simulink model "Simulation"  (R2019b)
settings: Solver=ode45  StartTime=0.0  StopTime=40  MaxStep=0.2  RelTol=1e-3  EnableMultiTasking=on
model workspace (MAT data in the model file):
  g_density = 5
libraries: sm_stewart_platform_lib x8, sm_lib x2, nesl_utility x1
Description:
  | Stewart Platform
  | 
  | This model shows a Stewart platform manipulator that can track a
  | parameterized reference trajectory. The shape, size, and kinematics of
  | the manipulator are highly configurable.
  | 
  | The reference trajectory is
  | specified in 6-D pose space, and an inverse kinematics module
  | converts it into one through 6-D leg position space.  A generic PID
  | controller attempts to drive the manipulator along the desired
  | trajectory.
settings Model: FPTRunName=Active  Creator=MathWorks  LastModifiedBy=hakon
settings DataIOCC: LimitDataPoints=on  SaveFormat=Array  SignalLoggingSaveFormat=ModelDataLogs  ReturnWorkspaceOutputs=off
settings OptimizationCC: ExpressionDepthLimit=2147483647  LifeSpan=inf
settings DebuggingCC: UnderspecifiedInitializationDetection=Classic  MergeDetectMultiDrivingBlocksExec=none  SolverPrmCheckMsg=warning  FcnCallInpInsideContextMsg=warning  StateNameClashWarn=warning  SFUnexpectedBacktrackingDiag=warning  SFNoUnconditionalDefaultTransitionDiag=warning  SFExecutionAtInitializationDiag=none  ArithmeticOperatorsInVariantConditions=warning
settings HardwareCC: ProdBitPerPointer=32  ProdBitPerSizeT=32  ProdBitPerPtrDiffT=32  ProdLargestAtomicFloat=None  ProdIntDivRoundTo=Undefined  ProdEndianess=Unspecified  ProdWordSize=32  ProdHWDeviceType=32-bit Generic
settings ModelReferenceCC: PropagateSignalLabelsOutOfModel=off
settings SFSimCC: SimUseLocalCustomCode=off  CustomCodeUndefinedFunction=UseInterfaceOnly
settings RTWCC: RTWUseLocalCustomCode=off
settings CodeAppCC: StateflowObjectComments=on
settings GRTTargetCC: TargetLangStandard=C89/C90 (ANSI)  GeneratePreprocessorConditionals=Disable all  CombineOutputUpdateFcns=off  GRTInterface=on
settings ConfigComp: CovMetricSettings=dw  CovHtmlReporting=on  CovSaveCumulativeToWorkspaceVar=on  CovSaveSingleToWorkspaceVar=on  CovExternalEMLEnable=off
settings SimscapeCC: SimscapeNormalizeSystem=off  SimscapeLogDataHistory=15000
settings ConfigurationSet: Description=SimMechanics 2G

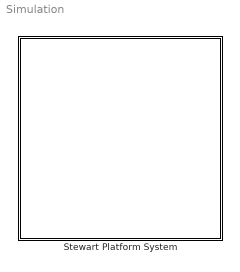
== system Simulation ==
  Stewart Platform System : Subsystem  mask(Stewart Platform System){base_rad=30, base_thick=5, platform_rad=20, platform_thick=0.5, hex_skew=-0.25, upper_leg_len=8, lower_leg_len=8, leg_rad=2, collar_thick=0.5, gripper_height=30, claw_length=8, claw_width=3, claw_thick=1, end_eff_base_thick=2, flange_len=2.3, flange_width=1.75, flange_thick=.8, ic_R=eye(3), ic_d=[0 0 15]', Kp=600, Ki=60, Kd=10}
      mask prompts: base_rad "Base Radius  (cm)"; base_thick "Base Thickness (cm)"; platform_rad "Platform Radius (cm)"; platform_thick "Platform Thickness (cm)"; hex_skew "Hexagon Skew"; upper_leg_len "Upper Leg Length (cm)"; lower_leg_len "Lower Leg Length (cm)"; leg_rad "Leg Radius (cm)"; collar_thick "Collar Thickness (cm)"; gripper_height "Gripper Height (cm)"; claw_length "Claw Length (cm)"; claw_width "Claw Width (cm)"; claw_thick "Claw Thickness (cm)"; end_eff_base_thick "Base Thickness (cm)"; flange_len "Flange Length (cm)"; flange_width "Flange Width (cm)"; flange_thick "Flange Thickness (cm)"; ic_R "Rotation Matrix [3 x 3]"; ic_d "Displacement Vector (cm) [3 x 1]"; Kp "Controller Proportional Gain (N / cm)"; Ki "Controller Integral Gain (N / (cm s))"; Kd "Controller Derivative Gain (N / (cm / s)))"
      mask help:
      | Models a complete Stewart platform manipulator system.  The system can be driven to position and orient a special gripper frame according to specified trajectories.
      |
      | The system comprises a mechanical manipulator, an inverse kinematics module, and a control system.
      mask init:
      | params = struct( ...
      |     'base_thick',        base_thick,     ...
      |     'base_radius',       base_rad,       ...
      |     'platform_thick',    platform_thick, ...
      |     'platform_radius',   platform_rad,   ...
      |     'skew',              hex_skew,       ...
      |     'flange_length',     flange_len,     ...
      |     'flange_width',      flange_width,   ...
      |     'flange_thick',      flange_thick,   ...
      |     'leg_radius',        leg_rad,        ...
      |     'upper_leg_length',  upper_leg_len,  ...
      |     'lower_leg_length',  lower_leg_len,  ...
      |     'gripper_height',    gripper_height  ...
      |     );
      | 
      | [B, P, nom_length] = sm_stewart_platform_setup(params);
      | 
      | lengths = sm_stewart_platform_ik(B, P, nom_length, ic_R, ic_d);
      mask Help:
      | A <em>Stewart Platform System</em> models a complete Stewart platform manipulator system.  The system can be driven to position and orient a special gripper frame according to specified trajectories.
      | 
      | <h3>Subsystems</h3>
      | 
      | A Stewart platform system comprises three primary subsystems:
      | 
      | <ol>
      | 
      | <li><b>Manipulator</b> The manipulator is the Simscape Multibody subsystem describing the mechanical structure of the Stewart platform.  The manipulator contains two hexagonal plates, a lower base plate and an upper platform plate, connected by six articulated legs.  The base plate is anchored to the world frame, and the platform plate is controlled to position and orient the gripper frame. The manipulator component provides sensing and actuation signals to interface to a controller.
      | 
      |   The manipulator is highly parameterized.  Most parameters of the Stewart platform system are physical lengths and other parameters that control the shapes and sizes of the components of the manipulator. By varying these parameters, a wide range of Stewart platform manipulators can be realized.
      | 
      | <li><b>Inverse Kinematics (IK) Module</b> The inverse kinematics module is a pure Simulink subsystem that maps time-varying signals describing the desired position and orientation of the gripper frame into time-varying scalar signals specifying the positions and velocities of the prismatic primitives of the leg joints.  This is an essential component of a complete Stewart platform system because the user of the system typically expresses a desired trajectory in the 6-D space of positions and orientations of the gripper frame, but the manipulator control is simplest in the 6-D space of leg joint positions. The IK module forms the bridge between these two spaces.
      | 
      |   The mathematics performed within the IK module is heavily dependent on the physical parameters that determine the shape and size of the manipulator itself.  Most of the parameters that govern the manipulator are also used within the IK module.
      | 
      | <li><b>Control System</b> The control system is a pure Simulink subsystem that attempts to drive the gripper frame along its desired trajectory by controlling the positions of the prismatic primitives of the leg joints. It uses a standard PID control scheme, with gains specified by Stewart platform system parameters.  The control uses no information about the forward or inverse kinematics of the platform; it simply tries to drive a point along a trajectory in 6-D space.
      | 
      |   The controller takes both the desired and actual leg position vectors and the first derivatives of these quantities.  It generates a 6-D commanded force output that can be used to drive the six leg lengths to thei desired values.
      | 
      |   Because the size and shape of the Stewart platform manipulator can vary significantly depending on the parameter settings, the controller gains may need to be adjusted in order to control the manipulator to the desired trajectory.
      | 
      | </ol>
      | 
      | <h3>Base and Platform Plates</h3>
      | 
      | The <em>Plates</em> tab parameters specify the geometry of the base and platform hexagon plates of the Stewart platform manipulator.  See the documentation of the <em>Hexagon Plate</em> library block for details.
      | 
      | <ul>
      | 
      | <li> <b>Base Radius</b> The radius of the base plate.  The vertices of the hexagonal cross section all lie on a circle of this radius.
      | 
      | <li> <b>Base Thickness</b> The thickness of the base plate.
      | 
      | <li> <b>Platform Radius</b> The radius of the platform plate.  The vertices of the hexagonal cross section all lie on a circle of this radius.
      | 
      | <li> <b>Platform Thickness</b> The thickness of the platform plate.
      | 
      | <li> <b>Hexagon Skew</b> The common skew factor of the base and platform plates. This value, in the range (-0.5, +0.5), determines the shape of the three-fold symmetric hexagons.  A zero skew factor produces regular hexagons.  As the skew factor magnitude increases, the hexagons become more triangular.
      | 
      | </ul>
      | 
      | <h3>Legs</h3>
      | 
      | The <em>Legs</em> tab parameters specify the common geometry of the six legs of the Stewart platform manipulator.  See the documentation of the <em>Leg</em> library block for details.
      | 
      | <ul>
      | 
      | <li> <b>Upper Leg Length</b> The length of the upper leg, including its end collars.
      | 
      | <li> <b>Lower Leg Length</b> The length of the lower leg, including its end collars.
      | 
      | <li> <b>Leg Radius</b> The common radius of the upper and lower leg segments. Each segment's cross section is a regular hexagon inscribed in a circle of this radius.
      | 
      | <li> <b>Collar Thickness</b> The thickness of the hexagonal collars adjoined to the ends of each leg segment.
      | 
      | </ul>
      | 
      | <h3>End Effector</h3>
      | 
      | The <em>End Eff</em> tab parameters specify the geometry of the end effector attached to the platform plate of the Stewart platform manipulator. See the documentation of the <em>End Effector</em> block within the <em>Manipulator</em> subsystem for details.
      | 
      | <ul>
      | 
      | <li> <b>Gripper Height</b> The vertical distance from the origin of the gripper frame to the top surface of the movable platform plate.
      | 
      | <li> <b>Claw Length</b> The length (height) of the trapezoidal claws of the gripper.
      | 
      | <li> <b>Claw Width</b> The width of the trapezoidal claws of the gripper where they attach to the gripper base.
      | 
      | <li> <b>Claw Thickness</b> The thickness of the trapezoidal claws of the gripper.
      | 
      | <li> <b>Base Thickness</b> The thickness of the triangular gripper base.
      | 
      | </ul>
      | 
      | <h3>Flanges</h3>
      | 
      | The <em>Flanges</em> tab parameters specify the common geometry of the 48 flanges attached to the hexagonal plates and legs of the Stewart platform manipulator.  Each of the 12 universal joints is supported by four flanges.  See the documentation of the <em>Flange</em> library block for details.
      | 
      | <ul>
      | 
      | <li> <b>Flange Length</b> The length of the rectangular prism portion of the flanges.
      | 
      | <li> <b>Flange Width</b> The width of the rectangular prism portion of the flanges.
      | 
      | <li> <b>Flange Thickness</b> The thickness of the flanges.
      | 
      | </ul>
      | 
      | <h3>Initial Conditions</h3>
      | 
      | The <em>IC</em> tab parameters specify the initial conditions of the Stewart Platform manipulator for simulation.  Specifically, these specify the <em>position</em> of the manipulator; the simulation always starts from a rest (zero velocity) state.
      | 
      | The initial position is defined by specifying pose of the gripper frame relative to the world frame.  This is typically a convenient parameterization for a user of the manipulator.  The world frame is also the reference frame of the manipulator base plate.  This is a frame with origin at the center of the manipulator base (which is in its interior), and with z-axis pointed directly upward.
      | 
      | An Update Diagram (Ctrl-D) operation will attempt to assemble the manipulator in the specified initial position.  Some initial positions may be incompatible with the kinematics of the manipulator, based on other parameter settings.  In such cases, the assembly will fail.
      | 
      | Also note that if the initial position differs significantly from the desired trajectory (specified through the input signal ports) at time zero, the manipulator's motion may be subject to large transients at the start of simulation.
      | 
      | <ul>
      | 
      | <li> <b>Rotation Matrix</b> The rotation matrix mapping directions in the gripper frame to directions in the world frame.  This should be a 3 x 3 orthogonal matrix determinant +1.  The columns of this matrix are the canonical i, j, and k unit vectors of the gripper frame resolved in world frame coordinates.
      | 
      | <li> <b>Displacement Vector</b> The location of the origin of the gripper frame in world frame coordinates.  This should be a 3 x 1 column vector.  The z-coordinate should generally be positive, on the order of the nominal lengths of the legs.
      | 
      | </ul>
      | 
      | If the rotation matrix is the identity and the x- and y-coordinates of the displacement vector are zero, the initial configuration of the manipulator will be symmetric with all leg positions equal.
      | 
      | <h3>Controller Gains</h3>
      | 
      | The <em>Control</em> tab parameters specify the gains of the internal controller used to control the manipulator's pose according to a specified trajectory.  The controller uses a generic PID control scheme.  The gains may need to be adjusted to be appropriate if the parameters governing the size and kinematics of the manipulator are changed significantly.
      | 
      | See the documentation of the <em>Controller</em> subsystem for details.
      | 
      | <ul>
      | 
      | <li> <b>Controller Proportional Gain</b> The proportional (P) gain of the internal PID controller.
      | 
      | <li> <b>Controller Integral Gain</b> The integral (I) gain of the internal PID controller.
      | 
      | <li> <b>Controller Derivative Gain</b> The derivative (D) gain of the internal PID controller.
      | 
      | </ul>
      | 
      | 
      | 
      | <h3>Ports</h3>
      | 
      | <ul>
      | 
      | <li><b>d</b> The desired displacement vector of the gripper frame relative to the world frame as a signal input.  This value should be a 3 x 1 vector in units of centimeters.  It specifies the desired origin of the gripper frame in world frame coordinates as a function of time.  This signal is analogous to the <em>Displacement Vector</em> on the <em>IC</em> parameter tab.
      | 
      | <li><b>R</b> The desired rotation matrix from the gripper frame to the world frame as a signal input.  This value should be a 3 x 3 orthogonal matrix with +1 determinant.  The columns of this matrix are the canonical i, j, and k unit vectors of the gripper frame resolved in world frame coordinates, specified as functions of time.  This signal is analogous to the <em>Rotation Matrix</em> on the <em>IC</em> parameter tab.
      | 
      | <li><b>d'</b> The first time derivative of the desired displacement vector of the gripper frame relative to the world frame as a signal input.  This value should be the first time derivative of the signal provided on the <em>d</em> port: a 3 x 1 vector in units of centimeters/second. It specifies the velocity of the origin of the gripper frame in  world frame coordinates as a function of time.
      | 
      | <li><b>R'</b> The first time derivative of the desired rotation matrix from the gripper frame to the world frame as a signal input.  This value should be the first time derivative of the signal provided on the <em>R</em> port: a 3 x 3 matrix.
      | 
      | <li><b>Pos</b> The position of the gripper with respect to the world frame as a 3 x 1 position vector in units of centimeters.
      | </ul>
      | 
      | <!--  LocalWords:  Eff IC Ctrl IK
      |  -->
      mask Display:
      | image(imread('sm_stewart_platform_system.png'))
      | color('yellow')
      | port_label('Input', 1, 'd')
      | port_label('Input', 2, 'R')
      | port_label('Input', 3, 'd''')
      | port_label('Input', 4, 'R''')
      | port_label('Output', 1, 'Pos')

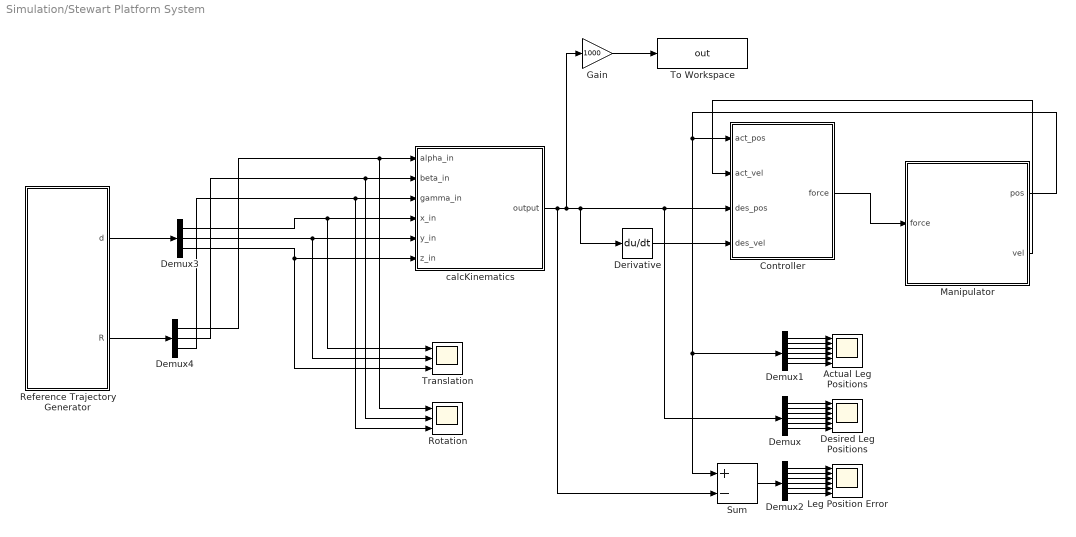
== system Simulation/Stewart Platform System ==
  Actual Leg Positions : Scope  NumInputPorts=6
  Controller : Subsystem  mask(PID Controller){Kp=Kp, Ki=Ki, Kd=Kd}
      mask prompts: Kp "Proportional Gain"; Ki "Integral Gain"; Kd "Derivative Gain"
      mask help:
      | Generates an actuation output based on a desired trajectory and an actual trajectory, using a generic proportional-integral-derivative (PID) control law.  The three control gains are specified through parameters.
      |
      | Both the desired and actual trajectories are specified by separate position and velocity input signals.  The controller is generic and can control to trajectories through state spaces of arbitrary dimension; the only requirement is that all four inputs have the same dimension.
      mask Help:
      | A <em>PID Controller</em> generates an actuation output based on a desired trajectory and an actual trajectory, using a generic proportional-integral-derivative (PID) control law.  The three control gains are specified through parameters.
      | 
      | Both the desired and actual trajectories are specified by separate position and velocity input signals.  The controller is generic and can control to trajectories through state spaces of arbitrary dimension; the only requirement is that all four inputs have the same dimension.
      | 
      | This block is not specific to the Stewart platform and could serve in any general purpose control library.  For the Stewart platform application, the trajectories are all through the 6-D leg-position space.
      | 
      | <h3>Gains</h3>
      | 
      | The parameters specify the gains of the controller.
      | 
      | <ul>
      | 
      | <li> <b>Proportional Gain</b> The gain that determines the strength of the control actuation in response to current deviations between actual and desired positions.  This affects the responsiveness of the controller but can lead to instability if set too high.
      | 
      | <li> <b>Integral Gain</b> The gain that determines the strength of the control actuation in response to deviations between actual and desired positions that persist over time.  A nonzero integral term is often necessary to avoid <em>droop</em> (steady-state error).  Higher values reduce the transient response of the controller but can cause overshoot in the controlled position.
      | 
      | <li> <b>Derivative Gain</b> The gain that determines the strength of the control actuation in response to the derivative of the deviations between actual and desired positions.  This is a damping component used to reduce overshoot in the controlled position; the tradeoff is that it reduces the transient response of the controller.  Higher values increase the stiffness of the system and can lead to instability.
      | 
      | </ul>
      | 
      | 
      | <h3>Ports</h3>
      | 
      | <ul>
      | 
      | <li> <b>act_pos</b> The current actual position of the plant.
      | 
      | <li> <b>act_pos</b> The current actual velocity of the plant.  This should be the time derivative of the <em>act_pos</em> signal.
      | 
      | <li> <b>des_pos</b> The current desired position of the plant.
      | 
      | <li> <b>des_pos</b> The current desired velocity of the plant.  This should be the time derivative of the <em>des_pos</em> signal.
      | 
      | </ul>
  Demux : Demux  Outputs=6
  Demux1 : Demux  Outputs=6
  Demux2 : Demux  Outputs=6
  Demux3 : Demux  Outputs=3
  Demux4 : Demux  Outputs=3
  Derivative : Derivative
  Desired Leg Positions : Scope  NumInputPorts=6
  Gain : Gain  Gain=1000
  Leg Position Error : Scope  NumInputPorts=6
  Manipulator : Subsystem  mask(Stewart Platform Manipulator){}
      mask help: Models the mechanical portion of a complete Stewart platform manipulator system: the manipulator itself. Almost all of the Simscape Multibody blocks of the full system are contained in the manipulator subsystem.
      mask Help:
      | A <em>Stewart Platform Manipulator</em> models the mechanical portion of a complete Stewart platform manipulator system: the manipulator itself.  Almost all of the Simscape Multibody blocks of the full system are contained in the manipulator subsystem.
      | 
      | The manipulator subsystem exposes two frames: the world frame, to which the base is anchored, and the gripper frame, which is the frame at the distil end of the end effector.  Typically, a user wants to control the manipulator transformation, which is the 3-D rigid transformation from the gripper frame to the world frame.
      | 
      | The manipulator subsystem has no internal control.  However, it reports the positions and velocities of the prismatic primitives of all six cylindrical leg joints as output signals and takes the actuation forces to be applied to these primitives as input signals.  When connected to an appropriate controller, these signals are sufficient to provide any of a variety of control schemes for the manipulator.
      | 
      | <h3>Parameterization</h3>
      | 
      | The manipulator is highly parameterized.  Most of the physical dimensions of its component pieces can be controlled via parameters.  These parameters are all defined in the containing <em>Stewart Platform System</em>.  The manipulator's parameters are inherited from that block; they are not defined explicitly in this block's mask.  The parameters are also needed for the <em>Stewart Platform Inverse Kinematics</em> block.
      | 
      | See the documentation of the <em>Stewart Platform System</em> block for details.
      | 
      | <h3>Ports</h3>
      | 
      | <ul>
      | 
      | <li> <b>gripper</b> The gripper frame.  This frame is fixed at the distil end of the end effector attached to the platform plate of the Stewart platform manipulator.  It is identified with a frame glyph in the visualization of the manipulator.  Typically, a user of the manipulator wants to control the pose of this frame, with respect to a reference frame such as world.
      | 
      | <li> <b>world</b> The world frame.  This is also the reference frame of the base plate of the Stewart platform manipulator, which is rigidly attached to the world frame.
      | 
      | <li><b>pos</b> The positions of the prismatic primitives of the six leg joints as a 6 x 1 output signal in units of centimeters.
      | 
      | <li><b>vel</b> The velocities of the prismatic primitives of the six leg joints as a 6 x 1 output signal in units of centimeters/second.
      | 
      | <li><b>force</b> The actuation forces applied to the prismatic primitives of the six leg joints as a 6 x 1 input signal in units of Newtons.
      | 
      | </ul>
      | 
      | <!--  LocalWords:  Eff IC Ctrl pos vel
      |  -->
      mask Display:
      | image(imread('sm_stewart_platform_manipulator.png'))
      | color('white')
      | port_label('LConn', 1, 'world')
      | port_label('RConn', 1, 'gripper')
      | color('yellow')
      | port_label('Input', 1, 'force')
      | port_label('Output', 1, 'pos')
      | port_label('Output', 2, 'vel')
  Reference Trajectory Generator : Subsystem
  Rotation : Scope  NumInputPorts=3
  Sum : Sum  Inputs=+-
  To Workspace : ToWorkspace  VariableName=out  SaveFormat=Timeseries  SampleTime=-1
  Translation : Scope  NumInputPorts=3
  calcKinematics : MATLAB Function  TreatAsAtomicUnit=on
  wires:
  Manipulator/2(vel) -> Controller/2(act_vel)
  Demux/1 -> Desired Leg Positions/1
  Demux/2 -> Desired Leg Positions/2
  Demux/3 -> Desired Leg Positions/3
  Demux/4 -> Desired Leg Positions/4
  Demux/5 -> Desired Leg Positions/5
  Demux/6 -> Desired Leg Positions/6
  Demux1/1 -> Actual Leg Positions/1
  Demux1/2 -> Actual Leg Positions/2
  Demux1/3 -> Actual Leg Positions/3
  Demux1/4 -> Actual Leg Positions/4
  Demux1/5 -> Actual Leg Positions/5
  Demux1/6 -> Actual Leg Positions/6
  Demux2/1 -> Leg Position Error/1
  Demux2/2 -> Leg Position Error/2
  Demux2/3 -> Leg Position Error/3
  Demux2/4 -> Leg Position Error/4
  Demux2/5 -> Leg Position Error/5
  Demux2/6 -> Leg Position Error/6
  Sum/1 -> Demux2/1
  Controller/1(force) -> Manipulator/1(force)
  Manipulator/1(pos) -> Controller/1(act_pos), Demux1/1, Sum/1
  calcKinematics/1(output) -> Sum/2, Gain/1, Derivative/1, Demux/1, Controller/3(des_pos)
  Derivative/1 -> Controller/4(des_vel)
  Reference Trajectory Generator/1(d) -> Demux3/1
  Demux3/2 -> Translation/2, calcKinematics/5(y_in)
  Demux3/3 -> Translation/3, calcKinematics/6(z_in)
  Reference Trajectory Generator/2(R) -> Demux4/1
  Demux4/1 -> Rotation/1, calcKinematics/1(alpha_in)
  Demux4/2 -> Rotation/2, calcKinematics/2(beta_in)
  Demux4/3 -> Rotation/3, calcKinematics/3(gamma_in)
  Demux3/1 -> Translation/1, calcKinematics/4(x_in)
  Gain/1 -> To Workspace/1

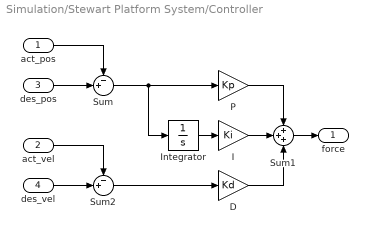
== system Simulation/Stewart Platform System/Controller ==
  act_pos : Inport
  act_vel : Inport  Port=2
  des_pos : Inport  Port=3
  des_vel : Inport  Port=4
  D : Gain  Gain=Kd  SaturateOnIntegerOverflow=on  OutDataTypeStr=Inherit: Same as input  ParamDataTypeStr=Inherit: Same as input
  I : Gain  Gain=Ki  SaturateOnIntegerOverflow=on  OutDataTypeStr=Inherit: Same as input  ParamDataTypeStr=Inherit: Same as input
  Integrator : Integrator  ZeroCross=off
  P : Gain  Gain=Kp  SaturateOnIntegerOverflow=on  OutDataTypeStr=Inherit: Same as input  ParamDataTypeStr=Inherit: Same as input
  Sum : Sum  Inputs=-+|  SaturateOnIntegerOverflow=on  InputSameDT=on  OutDataTypeStr=Inherit: Same as first input
  Sum1 : Sum  Inputs=+++  SaturateOnIntegerOverflow=on  InputSameDT=on  OutDataTypeStr=Inherit: Same as first input
  Sum2 : Sum  Inputs=-+|  SaturateOnIntegerOverflow=on  InputSameDT=on  OutDataTypeStr=Inherit: Same as first input
  force : Outport  VectorParamsAs1DForOutWhenUnconnected=off
  wires:
  Sum2/1 -> D/1
  D/1 -> Sum1/3
  Integrator/1 -> I/1
  P/1 -> Sum1/1
  I/1 -> Sum1/2
  Sum/1 -> P/1, Integrator/1
  act_pos/1 -> Sum/1
  des_pos/1 -> Sum/2
  Sum1/1 -> force/1
  act_vel/1 -> Sum2/1
  des_vel/1 -> Sum2/2

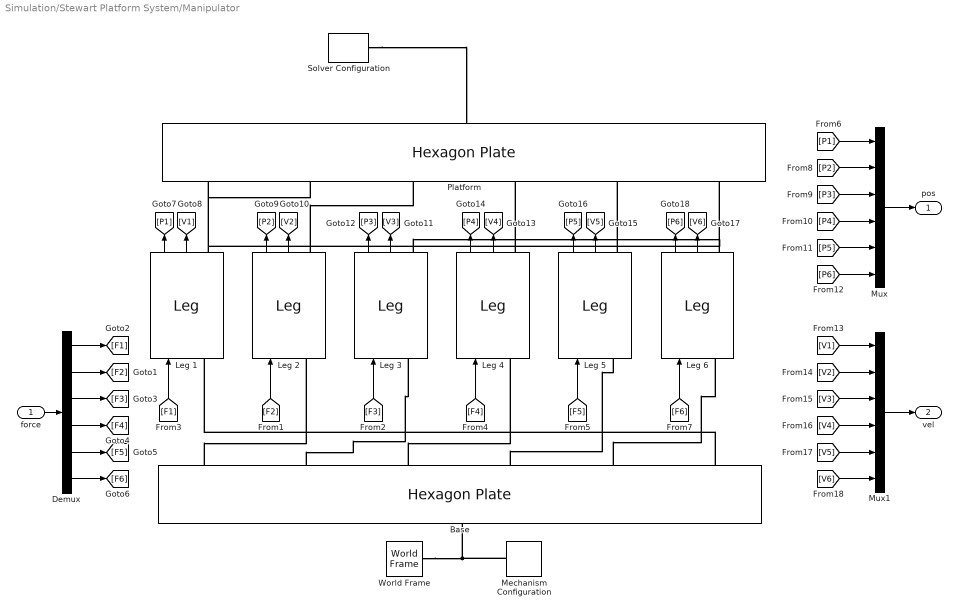
== system Simulation/Stewart Platform System/Manipulator ==
  force : Inport
  Base : sm_stewart_platform_lib/Hexagon Plate  kind=base  hex_rad=base_rad  hex_thick=base_thick  hex_skew=hex_skew  flange_sep=2 * leg_rad * cos(pi/6) - flange_thick  flange_len=flange_len  flange_width=flange_width  flange_thick=flange_thick  diffuse=[0.4 0.3 0.2 0.5]  specular=[0 0 0]  shininess=10
      settings: SourceProductName=Simscape Multibody  SourceProductBaseCode=MS
  Demux : Demux  Outputs=6
  Leg 1 : sm_stewart_platform_lib/Leg  upper_leg_len=upper_leg_len  lower_leg_len=lower_leg_len  rad=leg_rad  collar_thick=collar_thick  flange_len=flange_len  flange_width=flange_width  flange_thick=flange_thick  asm_offset=lengths(1)
      settings: SourceProductName=Simscape Multibody  SourceProductBaseCode=MS
  Leg 2 : sm_stewart_platform_lib/Leg  upper_leg_len=upper_leg_len  lower_leg_len=lower_leg_len  rad=leg_rad  collar_thick=collar_thick  flange_len=flange_len  flange_width=flange_width  flange_thick=flange_thick  asm_offset=lengths(2)
      settings: SourceProductName=Simscape Multibody  SourceProductBaseCode=MS
  Leg 3 : sm_stewart_platform_lib/Leg  upper_leg_len=upper_leg_len  lower_leg_len=lower_leg_len  rad=leg_rad  collar_thick=collar_thick  flange_len=flange_len  flange_width=flange_width  flange_thick=flange_thick  asm_offset=lengths(3)
      settings: SourceProductName=Simscape Multibody  SourceProductBaseCode=MS
  Leg 4 : sm_stewart_platform_lib/Leg  upper_leg_len=upper_leg_len  lower_leg_len=lower_leg_len  rad=leg_rad  collar_thick=collar_thick  flange_len=flange_len  flange_width=flange_width  flange_thick=flange_thick  asm_offset=lengths(4)
      settings: SourceProductName=Simscape Multibody  SourceProductBaseCode=MS
  Leg 5 : sm_stewart_platform_lib/Leg  upper_leg_len=upper_leg_len  lower_leg_len=lower_leg_len  rad=leg_rad  collar_thick=collar_thick  flange_len=flange_len  flange_width=flange_width  flange_thick=flange_thick  asm_offset=lengths(5)
      settings: SourceProductName=Simscape Multibody  SourceProductBaseCode=MS
  Leg 6 : sm_stewart_platform_lib/Leg  upper_leg_len=upper_leg_len  lower_leg_len=lower_leg_len  rad=leg_rad  collar_thick=collar_thick  flange_len=flange_len  flange_width=flange_width  flange_thick=flange_thick  asm_offset=lengths(6)
      settings: SourceProductName=Simscape Multibody  SourceProductBaseCode=MS
  Mechanism Configuration : sm_lib/Utilities/Mechanism Configuration  UniformGravity=Constant  GravityVector=[0 0 -9.81]  GravityUnits=m/s^2  LinearizationDelta=0.001
  Mux : Mux  Inputs=6
  Mux1 : Mux  Inputs=6
  Platform : sm_stewart_platform_lib/Hexagon Plate  kind=platform  hex_rad=platform_rad  hex_thick=platform_thick  hex_skew=hex_skew  flange_sep=2 * leg_rad * cos(pi/6) - flange_thick  flange_len=flange_len  flange_width=flange_width  flange_thick=flange_thick  diffuse=[.7 .7 .3 0.75]  specular=[.7 .7 .3 0.75]  shininess=90
      settings: SourceProductName=Simscape Multibody  SourceProductBaseCode=MS
  Solver Configuration : nesl_utility/Solver Configuration  PhysicalDomain=network_engine_domain  SubClassName=solver  LeftPortType=input  RightPortType=generic  Tones=[]  Harmonics=[]  SimulateNoise=off  Profile=off  UseLocalSampling=off  EnableSwitchedLinearOptims=on  FrequencyDomain=off  UseCCode=off  RelTol=0.001  AbsTol=1e-06  MinStep=1e-09  ToWorkspace=off  RevertToSquareIcSolve=off  NumHomotopyIterations=100  PhasorMode=off  PhasorModeNumHarmonics=1  DoDC=off  ResidualTolerance=1e-9  UseLocalSolver=off  LocalSolverChoice=NE_BACKWARD_EULER_ADVANCER  LocalSolverSampleTime=.001  DoFixedCost=off  MaxNonlinIter=3  MaxModeIter=2  LinearAlgebra=Sparse  EquationFormulation=NE_TIME_EF  DelaysMemoryBudget=1024  AutomaticFiltering=on  FilteringTimeConstant=0.001  PartitionStorageMethod=AS_NEEDED  PartitionMemoryBudget=1024  PartitionMethod=FAST
  World Frame : sm_lib/Frames and Transforms/World Frame
  pos : Outport  VectorParamsAs1DForOutWhenUnconnected=off
  vel : Outport  Port=2  VectorParamsAs1DForOutWhenUnconnected=off
  wires:
  Demux/1 -> [F1]
  Demux/2 -> [F2]
  Demux/3 -> [F3]
  Demux/4 -> [F4]
  Demux/5 -> [F5]
  Demux/6 -> [F6]
  [F1] -> Leg 1/1
  [F2] -> Leg 2/1
  [F3] -> Leg 3/1
  [F4] -> Leg 4/1
  [F5] -> Leg 5/1
  [F6] -> Leg 6/1
  force/1 -> Demux/1
  Leg 1/1 -> [P1]
  Leg 1/2 -> [V1]
  Leg 2/1 -> [P2]
  Leg 2/2 -> [V2]
  Leg 3/1 -> [P3]
  Leg 3/2 -> [V3]
  Leg 4/1 -> [P4]
  Leg 4/2 -> [V4]
  Leg 5/1 -> [P5]
  Leg 5/2 -> [V5]
  Leg 6/1 -> [P6]
  Leg 6/2 -> [V6]
  Mux/1 -> pos/1
  [P1] -> Mux/1
  [P2] -> Mux/2
  [P3] -> Mux/3
  [P4] -> Mux/4
  [P5] -> Mux/5
  [P6] -> Mux/6
  [V1] -> Mux1/1
  [V2] -> Mux1/2
  [V3] -> Mux1/3
  [V4] -> Mux1/4
  [V5] -> Mux1/5
  [V6] -> Mux1/6
  Mux1/1 -> vel/1
  connections:
  Solver Configuration/RConn1 -- Platform/LConn1
  Mechanism Configuration/RConn1 -- World Frame/RConn1 -- Base/LConn1
  Base/RConn1 -- Leg 2/LConn1
  Base/RConn2 -- Leg 3/LConn1
  Base/RConn3 -- Leg 4/LConn1
  Base/RConn4 -- Leg 5/LConn1
  Base/RConn5 -- Leg 6/LConn1
  Base/RConn6 -- Leg 1/LConn1
  Leg 1/RConn1 -- Platform/RConn2
  Leg 2/RConn1 -- Platform/RConn3
  Leg 3/RConn1 -- Platform/RConn4
  Leg 4/RConn1 -- Platform/RConn5
  Leg 5/RConn1 -- Platform/RConn6
  Leg 6/RConn1 -- Platform/RConn1

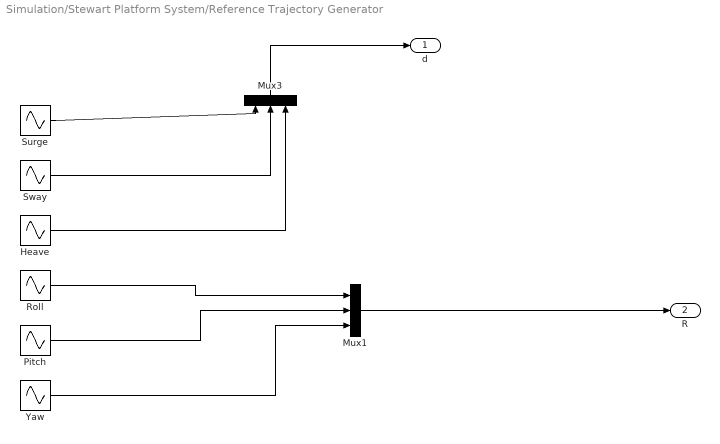
== system Simulation/Stewart Platform System/Reference Trajectory Generator ==
  Heave : Sin  Amplitude=0  Frequency=pi/10  SampleTime=0.1
  Mux1 : Mux  Inputs=3
  Mux3 : Mux  Inputs=3
  Pitch : Sin  Amplitude=pi/180*2  Frequency=pi * 3 / 10  Phase=-pi/2  SampleTime=0.01
  Roll : Sin  Amplitude=pi/180*2  Frequency=pi * 3 / 10  SampleTime=0.01
  Surge : Sin  Amplitude=0  Frequency=pi/10  SampleTime=0.1
  Sway : Sin  Amplitude=0  Frequency=pi/10  Phase=-pi/2  SampleTime=0.1
  Yaw : Sin  Amplitude=(pi/180)*2  Frequency=pi * 3 / 10  SampleTime=0.01
  d : Outport  VectorParamsAs1DForOutWhenUnconnected=off
  R : Outport  Port=2  VectorParamsAs1DForOutWhenUnconnected=off
  wires:
  Mux3/1 -> d/1
  Mux1/1 -> R/1
  Surge/1 -> Mux3/1
  Sway/1 -> Mux3/2
  Heave/1 -> Mux3/3
  Roll/1 -> Mux1/1
  Pitch/1 -> Mux1/2
  Yaw/1 -> Mux1/3

== matlab function Simulation/Stewart Platform System/calcKinematics ==
  data: alpha_in input; output output; beta_in input; gamma_in input; x_in input; y_in input; z_in input
function output  = calcKinematics(alpha_in, beta_in,gamma_in, x_in, y_in, z_in)

%Defining Roll Pitch Yaw angles
alpha = alpha_in;
beta = beta_in;
gamma = gamma_in;

%Defining rotation matrices in xyz
r_x = [1 0 0;
       0 cos(alpha) -sin(alpha);
       0 sin(alpha) cos(alpha)];

r_y = [cos(beta) 0 sin(beta);
       0 1 0;
       -sin(beta) 0 cos(beta)];

r_z = [cos(gamma) -sin(gamma) 0;
       sin(gamma) cos(gamma) 0;
       0 0 1];
   
%Definning desired positon vector
x = x_in;
y = y_in;
z = 212.21 + z_in + 5;

P = [x;y;z];


%Creating rotation marix
R = r_z*r_y*r_x;

%Coordinates relative to base frame for base spherical joints
a1_x = -142.28;
a1_y = -47.5;
a1_z = 0;
a1 = transpose([a1_x a1_y a1_z]);

a2_x = -112.28;
a2_y = -99.47;
a2_z = 0;
a2 = transpose([a2_x a2_y a2_z]);

a6_x = -30;
a6_y = 146.97;
a6_z = 0;
a6 = transpose([a6_x a6_y a6_z]);

a5_x = 30;
a5_y = 146.97;
a5_z = 0;
a5 = transpose([a5_x a5_y a5_z]);

a3_x = 112.28;
a3_y = -99.47;
a3_z = 0;
a3 = transpose([a3_x a3_y a3_z]);

a4_x = 142.28;
a4_y = -47.5;
a4_z = 0;
a4 = transpose([a4_x a4_y a4_z]);



%Coordinates relative to tool frame for top spherical joints
b1_x = -97.61;
b1_y = 21.72;
b1_z = 0;
b1 = transpose([b1_x b1_y b1_z]);

b6_x = -67.61;
b6_y = 73.68;
b6_z = 0;
b6 = transpose([b6_x b6_y b6_z]);

b2_x = -30;
b2_y = -95.39;
b2_z = 0;
b2 = transpose([b2_x b2_y b2_z]);

b3_x = 30;
b3_y = -95.39;
b3_z = 0;
b3 = transpose([b3_x b3_y b3_z]);

b5_x = 67.61;
b5_y = 73.68;
b5_z = 0;
b5 = transpose([b5_x b5_y b5_z]);

b4_x = 97.61;
b4_y = 21.72;
b4_z = 0;
b4 = transpose([b4_x b4_y b4_z]);


%Calculating leg vectors
s1 = P + R*b1 - a1;
s2 = P + R*b2 - a2;
s3 = P + R*b3 - a3;
s4 = P + R*b4 - a4;
s5 = P + R*b5 - a5;
s6 = P + R*b6 - a6;

%Calculating leg lenghts
l1 = sqrt(s1(1)^2 + s1(2)^2 + s1(3)^2);
l2 = sqrt(s2(1)^2 + s2(2)^2 + s2(3)^2);
l3 = sqrt(s3(1)^2 + s3(2)^2 + s3(3)^2);
l4 = sqrt(s4(1)^2 + s4(2)^2 + s4(3)^2);
l5 = sqrt(s5(1)^2 + s5(2)^2 + s5(3)^2);
l6 = sqrt(s6(1)^2 + s6(2)^2 + s6(3)^2);

%Calculating leg difference

d1 = l1 - 227;
d2 = l2 - 227;
d3 = l3 - 227;
d4 = l4 - 227;
d5 = l5 - 227;
d6 = l6 - 227;

output = [d1 ; d2 ; d3 ; d4 ; d5 ; d6];
end
